simulink model "simulation_pid"  (R2014b)
settings: Solver=ode45  StartTime=0.0  StopTime=10.0  RelTol=1e-3
PreLoadFcn:
  | simulation_consts;
undefined symbols (not defined in the file or in its folder): P, simulation_plot_tanks
libraries: simulink x4, simulink_need_slupdate x2
settings Model: Creator=cfppwin  LastModifiedBy=cfppwin

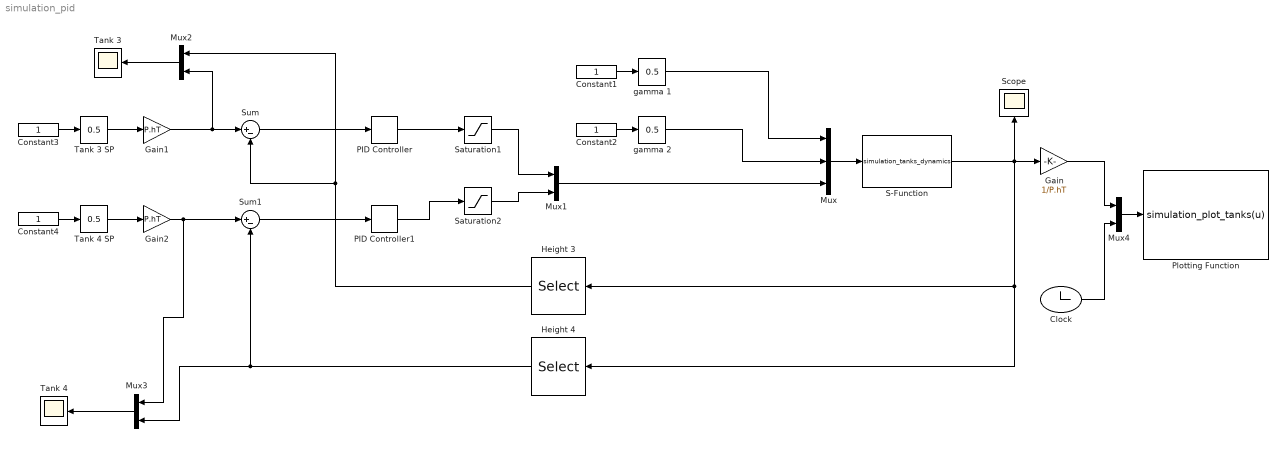
== system simulation_pid ==
  Clock : Clock
  Constant{1..4} (4 alike) : Constant
  Gain : Gain  Gain=1/P.hT
  Gain1 : Gain  Gain=P.hT
  Gain2 : Gain  Gain=P.hT
  Height 3 : Selector  InputPortWidth=4  Indices=3
  Height 4 : Selector  InputPortWidth=4  Indices=4
  Mux : Mux  Inputs=3
  Mux{1..4} (4 alike) : Mux  Inputs=2
  PID Controller : simulink_need_slupdate/PID Controller  P=.1  I=.0015  D=0
  PID Controller1 : simulink_need_slupdate/PID Controller  P=.1  I=.0015  D=0
  Plotting Function : MATLABFcn  MATLABFcn=simulation_plot_tanks(u)  OutputDimensions=0  SampleTime=0.1
  S-Function : S-Function  FunctionName=simulation_tanks_dynamics  Parameters=P  EnableBusSupport=off
  Saturation1 : Saturate  UpperLimit=1  LowerLimit=.001
  Saturation2 : Saturate  UpperLimit=1  LowerLimit=.001
  Scope : Scope
      settings: YMin=6  YMax=24
  Sum : Sum  Inputs=|+-
  Sum1 : Sum  Inputs=|+-
  Tank 3 : Scope
      settings: TimeRange=150  YMin=16  YMax=29
  Tank 3 SP : simulink/Math Operations/Slider Gain  low=0  gain=0.5  high=1
  Tank 4 : Scope
      settings: TimeRange=150  YMin=16  YMax=29  SaveName=ScopeData2
  Tank 4 SP : simulink/Math Operations/Slider Gain  low=0  gain=0.5  high=1
  gamma 1 : simulink/Math Operations/Slider Gain  low=0  gain=0.5  high=1
  gamma 2 : simulink/Math Operations/Slider Gain  low=0  gain=0.5  high=1
  wires:
  Constant2/1 -> gamma 2/1
  Constant1/1 -> gamma 1/1
  gamma 1/1 -> Mux/1
  S-Function/1 -> Scope/1, Height 3/1, Height 4/1, Gain/1
  Mux/1 -> S-Function/1
  Constant3/1 -> Tank 3 SP/1
  Constant4/1 -> Tank 4 SP/1
  Tank 4 SP/1 -> Gain2/1
  Tank 3 SP/1 -> Gain1/1
  Gain1/1 -> Mux2/2, Sum/1
  Gain2/1 -> Sum1/1, Mux3/1
  Sum/1 -> PID Controller/1
  Sum1/1 -> PID Controller1/1
  Height 3/1 -> Mux2/1, Sum/2
  Height 4/1 -> Sum1/2, Mux3/2
  PID Controller/1 -> Saturation1/1
  Saturation1/1 -> Mux1/1
  PID Controller1/1 -> Saturation2/1
  Saturation2/1 -> Mux1/2
  Mux2/1 -> Tank 3/1
  Mux3/1 -> Tank 4/1
  Mux4/1 -> Plotting Function/1
  Clock/1 -> Mux4/2
  Gain/1 -> Mux4/1
  Mux1/1 -> Mux/3
  gamma 2/1 -> Mux/2
